simulink library "tqd"  (R2021b)
settings: Solver=VariableStepAuto  StartTime=0.0  StopTime=10.0  RelTol=1e-3
undefined symbols (not defined in the file): ATQD_AfterTqMinGain_X_Deg, ATQD_APSCreepBaseTqD_X_kph, ATQD_APSCreepBaseTqD_Y_Deg, ATQD_APSCreepBaseTqR_X_kph, ATQD_APSCreepBaseTqR_Y_Deg, ATQD_APSCreepIterm_X_kph, ATQD_APSCreepIterm_Y_kph, ATQD_APSCreepPterm_X_kph, ATQD_APSCreepPterm_Y_kph, ATQD_APSDecReq_X_kph, ATQD_APSDecReq_Y_mps2, ATQD_APSDecReqCMD_X_kph, ATQD_APSDecReqTs_X_pct, ATQD_APSDecTimeGain_X_Deg, ATQD_APSDecTimeGain_Y_s, ATQD_APSReqLowSpd_X_Deg, ATQD_AutoHoldReleaseBPS_X_Deg, ATQD_AWDLoadTrqnsGain_X_kg, ATQD_AWDLoadTrqnsGain_Y_pct, ATQD_BOSEnBPSPosn_X_kph, ATQD_BOSMap_X_rpm, ATQD_BOSMap_Y_pct, ATQD_CreepBaseTqD_X_kph, ATQD_CreepBaseTqD_Y_Deg, ATQD_CreepBaseTqR_X_kph, ATQD_CreepBaseTqR_Y_Deg, ATQD_CreepBPSDisPosn_X_Deg, ATQD_CreepBPSDisPosnR_X_Deg, ATQD_CreepBPSEnPosn_X_Deg, ATQD_CreepBPSEnPosnR_X_Deg, ATQD_CreepDeltaTq_X_kph, ATQD_CreepIterm_X_kph, ATQD_CreepIterm_Y_kph, ATQD_CreepItermMaxLimit_X_pct, ATQD_CreepPreloadTime_X_kph, ATQD_CreepPreloadTq_X_kph, ATQD_CreepPreloadTq_Y_s, ATQD_CreepProtTq_X_Deg, ATQD_CreepPterm_X_kph, ATQD_CreepPterm_Y_kph, ATQD_CreepRrTqSpRat_X_rpm, ATQD_CreepRrTqSpRat_Y_Nm, ATQD_CreepTargetSpdD_X_pct, ATQD_CreepTargetSpdR_X_pct, ATQD_ECOTqMapD_X_rpm, ATQD_ECOTqMapD_Y_pct, ATQD_EMTqMapD_X_rpm, ATQD_EMTqMapD_Y_pct, ATQD_EOPDTqMapDCon_X_rpm, ATQD_EOPDTqMapDCon_Y_Deg, ATQD_EscapeModePedTq_X_pct, ATQD_EscapeModePedTq_Y_rpm, ATQD_EscapeModePedTqFr_X_pct, ATQD_EscapeModePedTqFr_Y_rpm, ATQD_EstInitVehWeight_X_c, ATQD_FAfterTqCMDGain_X_rpm, ATQD_FAfterTqCMDGain_Y_pct, ATQD_FrLossMAPLowV_X_rpm, ATQD_FrLossMAPLowV_Y_Nm, ATQD_FrMotActReduce_X_rpm ... (+772)
libraries: simulink x211, hcu_lib x179, tqr x3
(part 17 of 28)

== system tqd/TQD/TorqueDemand/TorqueModule/TqDistribution/New Torque Distribution ==
  note: Torque Distribution Calculation
  note: Fr/Rr Wheel Torqrue Determination
  note: Motor Output Torque Status Determination
  note: Rr/Fr Motor Enable Output Torque Detection
  VPMM_DrivetrainSelect_enum : Inport
  VTQD_CoordTqDem_Nm : Inport  Port=2
  VTQR_NoABSFEDUWhlTqReq_Nm : Inport  Port=3
  VTQR_FrTqZeroTransLowBound_Nm : Inport  Port=4
  VTQR_NoABSREDUWhlTqReq_Nm : Inport  Port=5
  VTQR_RrTqZeroTransUpBound_Nm : Inport  Port=6
  VINP_RrMotorAvailTq_Nm : Inport  Port=7
  VINP_RrRegenAvailTq_Nm : Inport  Port=8
  VINP_FrMotorAvailTq_Nm : Inport  Port=9
  VINP_FrRegenAvailTq_Nm : Inport  Port=10
  VTQD_RrPreloadTq_Nm : Inport  Port=11
  VTQD_FrPreloadTq_Nm : Inport  Port=12
  VTQD_PreLoadHold_flg : Inport  Port=13
  AND{,1..8} (9 alike) : Logic  AllPortsSameDT=off  OutDataTypeStr=boolean
  Abs{,1..3} (4 alike) : Abs
  Add : Sum
  Add{1..3,5} (4 alike) : Sum  Inputs=+-
  Add4 : Sum
  Constant{1..2,21,49} (4 alike) : Constant  Value=KTQD_TqDemEnRrTMOutpRgn_Nm
  Constant10 : Constant  Value=KTQD_TqDemEnFrTMOutpMotDev_Nm
  Constant11 : Constant  Value=TRUE
  Constant12 : Constant  Value=ENUM_DRIVETRAIN_AWD
  Constant13 : Constant  Value=TRUE
  Constant14 : Constant  Value=ENUM_DRIVETRAIN_FWD
  Constant{15,18,30,39} (4 alike) : Constant  Value=ENUM_TMENOUTPTQSTA_REAR
  Constant{16,24,31,38} (4 alike) : Constant  Value=ENUM_TMENOUTPTQSTA_FRONT
  Constant{17,19,25,35,43} (5 alike) : Constant  Value=ENUM_TMENOUTPTQSTA_BOTH
  Constant{20,22..23,26..28,33,41,51} (9 alike) : Constant  Value=ZERO_FLOAT
  Constant29 : Constant  Value=EPS
  Constant3 : Constant  Value=KTQD_TqDemEnRrTMOutpRgnDev_Nm
  Constant{32,36,40,44} (4 alike) : Constant  Value=KTQD_NewDistInitRate_rat
  Constant34 : Constant  Value=ONE_FLOAT
  Constant37 : Constant  Value=EPS
  Constant4 : Constant  Value=KTQD_TqDemEnRrTMOutpMot_Nm
  Constant42 : Constant  Value=ONE_FLOAT
  Constant45 : Constant  Value=KTQD_AWDRrRatio_rat_ovrdflg
  Constant46 : Constant  Value=KTQD_AWDRrRatio_rat_ovrdval
  Constant47 : Constant  Value=KTQD_AWDRrRatio_rat_ovrdflg
  Constant48 : Constant  Value=KTQD_AWDRrRatio_rat_ovrdval
  Constant5 : Constant  Value=KTQD_TqDemEnFrTMOutpRgn_Nm
  Constant50 : Constant  Value=KTQD_TqDemEnRrTMOutpRgnDev_Nm
  Constant6 : Constant  Value=ENUM_DRIVETRAIN_AWD
  Constant7 : Constant  Value=ENUM_DRIVETRAIN_RWD
  Constant8 : Constant  Value=KTQD_RrTMRgnOutpConSW_flg
  Constant9 : Constant  Value=KTQD_FrTMMotOutpConSW_flg
  Delay : Delay  DelayLength=1  InitialCondition=uint8(0)
      settings: AttributesFormatString=%<InitialCondition>
  Divide : Product  Inputs=*/
  Divide1 : Product  Inputs=*/
  Equal{,1..9} (10 alike) : RelationalOperator  Operator===  OutDataTypeStr=boolean  RndMeth=Simplest
  KTQD_FrTMTotalGearRatio_gain{,1..4} (5 alike) : Gain  Gain=KTQD_FrTMTotalGearRatio_gain
  KTQD_RrTMTotalGearRatio_gain{,1..5} (6 alike) : Gain  Gain=KTQD_RrTMTotalGearRatio_gain
  Max : MinMax  Function=max  Inputs=2
  Max1 : MinMax  Function=max  Inputs=2
  Min : MinMax  Inputs=2
  Min1 : MinMax  Function=max  Inputs=2
  NOT : Logic  Operator=NOT  AllPortsSameDT=off  OutDataTypeStr=boolean
  NOT2 : Logic  Operator=NOT  AllPortsSameDT=off  OutDataTypeStr=boolean
  OR{,1..7} (8 alike) : Logic  Operator=OR  AllPortsSameDT=off  OutDataTypeStr=boolean
  Relational Operator{,5,8..9,12..13,16} (7 alike) : RelationalOperator  OutDataTypeStr=boolean  RndMeth=Simplest
  Relational Operator1 : RelationalOperator  Operator=<  OutDataTypeStr=boolean  RndMeth=Simplest
  Relational Operator{3..4,10..11} (4 alike) : RelationalOperator  Operator===  OutDataTypeStr=boolean  RndMeth=Simplest
  Relational Operator{2,7,14..15} (4 alike) : RelationalOperator  Operator=<=  OutDataTypeStr=boolean  RndMeth=Simplest
  Relational Operator6 : RelationalOperator  Operator=<  OutDataTypeStr=boolean  RndMeth=Simplest
  Saturation : Saturate  UpperLimit=single(1)  LowerLimit=single(0)
      settings: AttributesFormatString=|
      | UpperLimit:%<UpperLimit>
      | LowerLimi:%<LowerLimit>
  Saturation Dynamic : simulink/Discontinuities/Saturation Dynamic  OutMin=[]  OutMax=[]  OutDataTypeStr=Inherit: Same as second input  OutDataType=fixdt(1, 16)  OutScaling=2^-10  DoSatur=off
  Saturation Dynamic1 : simulink/Discontinuities/Saturation Dynamic  OutMin=[]  OutMax=[]  OutDataTypeStr=Inherit: Same as second input  OutDataType=fixdt(1, 16)  OutScaling=2^-10  DoSatur=off
  Saturation Dynamic2 : simulink/Discontinuities/Saturation Dynamic  OutMin=[]  OutMax=[]  OutDataTypeStr=Inherit: Same as second input  OutDataType=fixdt(1, 16)  OutScaling=2^-10  DoSatur=off
  Saturation1 : Saturate  UpperLimit=single(1)  LowerLimit=single(0)
      settings: AttributesFormatString=|
      | UpperLimit:%<UpperLimit>
      | LowerLimi:%<LowerLimit>
  Switch{,1..21} (22 alike) : Switch  Criteria=u2 ~= 0
      settings: AttributesFormatString=%<Criteria>
  VTQD_TMEnOutpTqSta_enum : Outport
  VTQD_NewDistFrWhlTq_Nm : Outport  Port=2
  VTQD_NewDistRrWhlTq_Nm : Outport  Port=3
  VTQD_NewFrRatio_rat : Outport  Port=4
  VTQD_NewRrRatio_rat : Outport  Port=5
  wires:
  [VTQD_CoordTqDem_Nm] -> Add5/1
  Saturation Dynamic2/1 -> Switch21/3
  [VTQD_CoordTqDem_Nm] -> Add3/1
  Equal9/1 -> Switch17/2
  [VTQD_PreLoadHold_flg] -> Switch10/2
  Constant14/1 -> Relational Operator11/2
  NOT/1 -> AND6/2
  VTQD_FrPreloadTq_Nm/1 -> [VTQD_FrPreloadTq_Nm]
  Constant42/1 -> Switch16/1
  Relational Operator16/1 -> Switch21/2
  Constant12/1 -> Relational Operator10/2
  Constant41/1 -> Switch15/1
  Constant38/1 -> Equal7/2
  Constant10/1 -> Add1/2
  Abs/1 -> Max/1
  Switch17/1 -> Switch18/3
  Constant34/1 -> Switch12/1
  AND3/1 -> OR2/1
  Switch10/1 -> [VTQD_NewDistFrWhlTq_Nm]  "VTQD_NewDistFrWhlTq_Nm"
  Equal8/1 -> Switch15/2
  Equal3/1 -> OR5/2
  Relational Operator6/1 -> AND3/1
  [VTQD_FrPreloadTq_Nm] -> Switch10/1
  Constant8/1 -> Switch/2
  Constant1/1 -> Relational Operator1/2
  Constant40/1 -> Switch15/3
  [VTQD_PreLoadHold_flg] -> Switch18/2
  [VTQD_NewFrRatio_rat] -> VTQD_NewFrRatio_rat/1
  Constant31/1 -> Equal5/2
  Constant4/1 -> Relational Operator/2
  AND4/1 -> OR2/2
  Constant44/1 -> Switch18/1
  Constant48/1 -> Switch20/1
  Constant39/1 -> Equal8/2
  Equal1/1 -> OR4/2
  OR2/1 -> AND5/2
  OR6/1 -> Switch/3
  Saturation1/1 -> Switch17/1
  Switch11/1 -> Switch12/3
  [VTQR_NoABSFEDUWhlTqReq_Nm] -> Relational Operator2/1
  Constant2/1 -> Add/1
  OR3/1 -> [VTQD_FrTMEnOutpTq_flg]  "VTQD_FrTMEnOutpTq_flg"
  Constant43/1 -> Equal9/2
  [VTQD_CoordTqDem_Nm] -> Relational Operator1/1
  Switch16/1 -> Switch17/3
  VPMM_DrivetrainSelect_enum/1 -> [VPMM_DrivetrainSelect_enum]
  KTQD_RrTMTotalGearRatio_gain5/1 -> Saturation Dynamic2/3
  Switch15/1 -> Switch16/3
  [VTQD_TMEnOutpTqSta_enum] -> Equal9/1
  VINP_FrRegenAvailTq_Nm/1 -> [VINP_FrRegenAvailTq_Nm]
  Constant28/1 -> Saturation Dynamic1/3
  VINP_RrMotorAvailTq_Nm/1 -> [VINP_RrMotorAvailTq_Nm]
  Relational Operator3/1 -> AND1/1
  Abs2/1 -> Max1/1
  [VINP_RrMotorAvailTq_Nm] -> KTQD_RrTMTotalGearRatio_gain1/1
  Max1/1 -> Divide1/2
  Equal7/1 -> Switch16/2
  [VINP_FrRegenAvailTq_Nm] -> KTQD_FrTMTotalGearRatio_gain4/1
  [VTQD_TMEnOutpTqSta_enum] -> Equal5/1
  Abs3/1 -> Divide1/1
  [VTQD_CoordTqDem_Nm] -> Min1/1
  [VTQR_RrTqZeroTransUpBound_Nm] -> Relational Operator7/2
  Divide1/1 -> Saturation1/1
  Switch18/1 -> Switch20/3  "VTQD_InitNewFrRatio_rat"
  [VTQD_TMEnOutpTqSta_enum] -> Equal8/1
  [VINP_FrRegenAvailTq_Nm] -> KTQD_FrTMTotalGearRatio_gain2/1
  [VTQD_PreLoadHold_flg] -> Switch9/2
  [VTQD_CoordTqDem_Nm] -> Relational Operator/1
  Switch/1 -> AND/2
  Switch12/1 -> Switch13/3
  [VTQD_TMEnOutpTqSta_enum] -> Equal7/1
  AND6/1 -> Switch2/2
  Constant13/1 -> Switch/1
  [VTQD_NewDistFrWhlTq_Nm] -> Abs3/1
  [VTQD_CoordTqDem_Nm] -> Abs2/1
  Constant6/1 -> Relational Operator3/2
  Relational Operator5/1 -> AND2/2
  Constant37/1 -> Max1/2
  Switch20/1 -> [VTQD_NewFrRatio_rat]  "VTQD_NewFrRatio_rat"
  [VTQD_CoordTqDem_Nm] -> Relational Operator13/1
  VTQR_NoABSREDUWhlTqReq_Nm/1 -> [VTQR_NoABSREDUWhlTqReq_Nm]
  Switch14/1 -> Switch19/3  "VTQD_InitNewRrRatio_rat"
  Add/1 -> Relational Operator2/2
  Delay/1 -> Switch2/3
  Relational Operator7/1 -> AND3/2
  Constant45/1 -> Switch19/2
  [VTQD_TMEnOutpTqSta_enum] -> Equal4/1
  [VPMM_DrivetrainSelect_enum] -> Relational Operator10/1
  [VTQR_NoABSFEDUWhlTqReq_Nm] -> Relational Operator5/1
  Equal4/1 -> Switch12/2
  Equal/1 -> OR4/1
  AND1/1 -> OR1/2
  Constant7/1 -> Relational Operator4/2
  [VTQR_FrTqZeroTransLowBound_Nm] -> Relational Operator5/2
  Relational Operator/1 -> AND2/1
  AND/1 -> OR/2
  [VPMM_DrivetrainSelect_enum] -> Relational Operator4/1
  [VTQR_NoABSREDUWhlTqReq_Nm] -> Relational Operator7/1
  OR1/1 -> [VTQD_RrTMEnOutpTq_flg]  "VTQD_RrTMEnOutpTq_flg"
  [VTQR_NoABSREDUWhlTqReq_Nm] -> Relational Operator9/1
  [VTQD_FrTMEnOutpTq_flg] -> AND8/2
  AND5/1 -> OR3/2
  Relational Operator8/1 -> AND4/1
  [VINP_RrMotorAvailTq_Nm] -> KTQD_RrTMTotalGearRatio_gain/1
  Relational Operator9/1 -> Switch1/3
  [VTQD_TMEnOutpTqSta_enum] -> Equal2/1
  Constant11/1 -> Switch1/1
  Switch2/1 -> Switch3/3
  [VTQD_RrTMEnOutpTq_flg] -> NOT2/1
  Relational Operator15/1 -> OR7/2
  NOT2/1 -> AND7/1
  Constant17/1 -> Switch4/1
  VTQR_RrTqZeroTransUpBound_Nm/1 -> [VTQR_RrTqZeroTransUpBound_Nm]
  [VTQD_RrTMEnOutpTq_flg] -> AND6/1
  [VTQD_RrTMEnOutpTq_flg] -> AND8/1
  Equal5/1 -> Switch11/2
  [VTQD_TMEnOutpTqSta_enum] -> Equal/1
  OR/1 -> AND1/2
  AND2/1 -> OR/1
  Relational Operator2/1 -> OR6/1
  [VTQD_TMEnOutpTqSta_enum] -> Equal3/1
  Constant18/1 -> Equal/2
  AND7/1 -> Switch3/2
  [VTQD_CoordTqDem_Nm] -> Add2/1
  Constant9/1 -> Switch1/2
  Add1/1 -> Relational Operator9/2
  OR5/1 -> Switch7/2
  [VTQD_FrTMEnOutpTq_flg] -> NOT/1
  [VTQD_CoordTqDem_Nm] -> Relational Operator6/1
  Constant36/1 -> Switch14/1
  Switch3/1 -> Switch4/3
  Constant20/1 -> Relational Operator12/2
  Relational Operator11/1 -> OR3/1
  OR4/1 -> Switch5/2
  [VTQD_TMEnOutpTqSta_enum] -> Equal1/1
  AND8/1 -> Switch4/2
  [VINP_RrMotorAvailTq_Nm] -> KTQD_RrTMTotalGearRatio_gain2/1
  [VTQD_CoordTqDem_Nm] -> Relational Operator12/1
  Add2/1 -> Saturation Dynamic/2
  Constant25/1 -> Equal3/2
  KTQD_RrTMTotalGearRatio_gain/1 -> Add1/1
  Relational Operator12/1 -> Switch6/2
  [VTQD_TMEnOutpTqSta_enum] -> Equal6/1
  [VTQD_CoordTqDem_Nm] -> Min/1
  KTQD_RrTMTotalGearRatio_gain2/1 -> Min/2
  Switch6/1 -> Switch5/1
  Constant51/1 -> Saturation Dynamic2/1
  Constant35/1 -> Equal6/2
  Switch4/1 -> Delay/1, [VTQD_TMEnOutpTqSta_enum]  "VTQD_TMEnOutpTqSta_enum"
  Min/1 -> Switch6/1
  [VPMM_DrivetrainSelect_enum] -> Relational Operator11/1
  Constant3/1 -> Add/2
  Equal2/1 -> OR5/1
  [VINP_RrMotorAvailTq_Nm] -> KTQD_RrTMTotalGearRatio_gain4/1
  VINP_FrMotorAvailTq_Nm/1 -> [VINP_FrMotorAvailTq_Nm]
  VTQR_FrTqZeroTransLowBound_Nm/1 -> [VTQR_FrTqZeroTransLowBound_Nm]
  Relational Operator4/1 -> OR1/1
  KTQD_FrTMTotalGearRatio_gain4/1 -> Relational Operator16/1
  Min1/1 -> Switch8/3
  Constant26/1 -> Switch7/3
  KTQD_RrTMTotalGearRatio_gain4/1 -> Add3/2
  [VTQD_CoordTqDem_Nm] -> Relational Operator8/1
  [VINP_FrMotorAvailTq_Nm] -> KTQD_FrTMTotalGearRatio_gain1/1
  KTQD_FrTMTotalGearRatio_gain/1 -> Min1/2
  [VTQR_NoABSFEDUWhlTqReq_Nm] -> Relational Operator14/1
  Relational Operator13/1 -> Switch8/2
  Switch9/1 -> [VTQD_NewDistRrWhlTq_Nm]  "VTQD_NewDistRrWhlTq_Nm"
  Switch7/1 -> Switch10/3
  Switch5/1 -> Switch9/3
  [VPMM_DrivetrainSelect_enum] -> Relational Operator3/1
  Add3/1 -> Saturation Dynamic1/2
  Switch8/1 -> Switch7/1
  [VINP_RrRegenAvailTq_Nm] -> KTQD_RrTMTotalGearRatio_gain3/1
  KTQD_FrTMTotalGearRatio_gain2/1 -> Relational Operator15/2
  Constant5/1 -> Relational Operator6/2
  Constant16/1 -> Switch3/1
  Constant46/1 -> Switch19/1
  [VTQD_CoordTqDem_Nm] -> Abs/1
  [VTQD_RrPreloadTq_Nm] -> Switch9/1
  Constant27/1 -> Relational Operator13/2
  Max/1 -> Divide/2
  KTQD_RrTMTotalGearRatio_gain3/1 -> Saturation Dynamic/3
  Constant29/1 -> Max/2
  KTQD_FrTMTotalGearRatio_gain1/1 -> Saturation Dynamic1/1
  [VTQD_FrTMEnOutpTq_flg] -> AND7/2
  Constant19/1 -> Equal1/2
  Divide/1 -> Saturation/1
  Switch1/1 -> AND4/2
  Abs1/1 -> Divide/1
  Constant32/1 -> Switch11/3
  Relational Operator10/1 -> AND5/1
  [VINP_FrRegenAvailTq_Nm] -> Add4/1
  KTQD_RrTMTotalGearRatio_gain1/1 -> Relational Operator8/2
  Constant22/1 -> Switch5/3
  Saturation Dynamic1/1 -> Switch8/1
  [VTQD_NewDistRrWhlTq_Nm] -> Abs1/1
  Constant30/1 -> Equal4/2
  Constant23/1 -> Saturation Dynamic/1
  Constant33/1 -> Switch11/1
  Constant24/1 -> Equal2/2
  [VINP_FrRegenAvailTq_Nm] -> KTQD_FrTMTotalGearRatio_gain3/1
  [VINP_FrRegenAvailTq_Nm] -> KTQD_FrTMTotalGearRatio_gain/1
  Saturation/1 -> Switch13/1
  Add5/1 -> Saturation Dynamic2/2
  [VTQD_NewRrRatio_rat] -> VTQD_NewRrRatio_rat/1
  Constant15/1 -> Switch2/1
  Equal6/1 -> Switch13/2
  [VTQD_PreLoadHold_flg] -> Switch14/2
  [VINP_RrRegenAvailTq_Nm] -> KTQD_RrTMTotalGearRatio_gain5/1
  Constant49/1 -> Add5/2
  Constant47/1 -> Switch20/2
  Switch13/1 -> Switch14/3
  [VTQD_CoordTqDem_Nm] -> Relational Operator15/1
  KTQD_FrTMTotalGearRatio_gain3/1 -> Add2/2
  Saturation Dynamic/1 -> Switch21/1
  Switch21/1 -> Switch6/3
  VTQD_PreLoadHold_flg/1 -> [VTQD_PreLoadHold_flg]
  VINP_RrRegenAvailTq_Nm/1 -> [VINP_RrRegenAvailTq_Nm]
  Constant50/1 -> Add4/2
  Add4/1 -> Relational Operator14/2
  OR7/1 -> AND/1
  Relational Operator14/1 -> OR6/2
  Switch19/1 -> [VTQD_NewRrRatio_rat]  "VTQD_NewRrRatio_rat"
  VTQR_NoABSFEDUWhlTqReq_Nm/1 -> [VTQR_NoABSFEDUWhlTqReq_Nm]
  [VTQD_NewDistFrWhlTq_Nm] -> VTQD_NewDistFrWhlTq_Nm/1
  VTQD_RrPreloadTq_Nm/1 -> [VTQD_RrPreloadTq_Nm]
  Relational Operator1/1 -> OR7/1
  [VTQD_NewDistRrWhlTq_Nm] -> VTQD_NewDistRrWhlTq_Nm/1
  Constant21/1 -> Relational Operator16/2
  [VTQD_TMEnOutpTqSta_enum] -> VTQD_TMEnOutpTqSta_enum/1
  VTQD_CoordTqDem_Nm/1 -> [VTQD_CoordTqDem_Nm]

== system tqd/TQD/TorqueDemand/TorqueModule/TqDistribution/RWD_Ratio ==
  Action Port : ActionPort
  Constant : Constant  Value=ONE_FLOAT
  Constant1 : Constant  Value=ZERO_FLOAT
  VTQD_FrRatio_RWD : Outport
  VTQD_RrRatio_RWD : Outport  Port=2
  wires:
  Constant1/1 -> VTQD_FrRatio_RWD/1
  Constant/1 -> VTQD_RrRatio_RWD/1

== system tqd/TQD/TorqueDemand/Signal_convert/SWC2_Subsystem/Big Mike Combo/Combo Key Detection ==
  TASK_TIME_10_MS : Inport
  VSCP_ComboKeyEn_flg : Inport  Port=2
  VSCP_ComboKeyReset_flg : Inport  Port=3
  VSCP_ComboKey_enum : Inport  Port=4
  VSCP_ComboKeyEnter_flg : Inport  Port=5
  VSCP_StreetFightModeOff_flg : Inport  Port=6
  DiagnosisOff Mode : Subsystem
  Engineering Mode : Subsystem
  Exhibition Mode : Subsystem
  Manufacture Mode : Subsystem
  Street Fight Mode : Subsystem
  VSCP_StreetFightMode_flg : Outport
  VSCP_EngineeringMode_flg : Outport  Port=2
  VSCP_ManufactureMode_flg : Outport  Port=3
  VSCP_ExhibitionMode_flg : Outport  Port=4
  VSCP_DiagnosisOffMode_flg : Outport  Port=5
  wires:
  [VSCP_DiagnosisOffMode_flg] -> VSCP_DiagnosisOffMode_flg/1
  DiagnosisOff Mode/1(VSCP_DiagnosisOffMode_flg) -> [VSCP_DiagnosisOffMode_flg]
  [VSCP_ComboKey_enum] -> DiagnosisOff Mode/4(VSCP_ComboKey_enum)
  [VSCP_ComboKeyEnter_flg] -> DiagnosisOff Mode/5(VSCP_ComboKeyEnter_flg)
  [TASK_TIME_10_MS] -> DiagnosisOff Mode/1(TASK_TIME_10_MS)
  [VSCP_ComboKeyReset_flg] -> DiagnosisOff Mode/3(VSCP_ComboKeyReset_flg)
  [VSCP_StreetFightModeOff_flg] -> DiagnosisOff Mode/6(VSCP_StreetFightModeOff_flg)
  [VSCP_ComboKeyEn_flg] -> DiagnosisOff Mode/2(VSCP_ComboKeyEn_flg)
  [VSCP_ExhibitionMode_flg] -> VSCP_ExhibitionMode_flg/1
  [VSCP_ManufactureMode_flg] -> VSCP_ManufactureMode_flg/1
  Exhibition Mode/1(VSCP_ExhibitionMode_flg) -> [VSCP_ExhibitionMode_flg]
  [VSCP_ComboKeyEn_flg] -> Exhibition Mode/2(VSCP_ComboKeyEn_flg)
  [VSCP_StreetFightModeOff_flg] -> Exhibition Mode/6(VSCP_StreetFightModeOff_flg)
  [VSCP_ComboKeyReset_flg] -> Exhibition Mode/3(VSCP_ComboKeyReset_flg)
  [TASK_TIME_10_MS] -> Exhibition Mode/1(TASK_TIME_10_MS)
  [VSCP_ComboKeyEnter_flg] -> Exhibition Mode/5(VSCP_ComboKeyEnter_flg)
  [VSCP_ComboKey_enum] -> Exhibition Mode/4(VSCP_ComboKey_enum)
  Manufacture Mode/1(VSCP_ManufactureMode_flg) -> [VSCP_ManufactureMode_flg]
  [VSCP_ComboKey_enum] -> Manufacture Mode/4(VSCP_ComboKey_enum)
  [VSCP_ComboKeyEnter_flg] -> Manufacture Mode/5(VSCP_ComboKeyEnter_flg)
  [TASK_TIME_10_MS] -> Manufacture Mode/1(TASK_TIME_10_MS)
  [VSCP_ComboKeyReset_flg] -> Manufacture Mode/3(VSCP_ComboKeyReset_flg)
  [VSCP_StreetFightModeOff_flg] -> Manufacture Mode/6(VSCP_StreetFightModeOff_flg)
  [VSCP_ComboKeyEn_flg] -> Manufacture Mode/2(VSCP_ComboKeyEn_flg)
  [VSCP_EngineeringMode_flg] -> VSCP_EngineeringMode_flg/1
  [VSCP_StreetFightMode_flg] -> VSCP_StreetFightMode_flg/1
  [VSCP_ComboKeyEn_flg] -> Engineering Mode/2(VSCP_ComboKeyEn_flg)
  [VSCP_StreetFightModeOff_flg] -> Engineering Mode/6(VSCP_StreetFightModeOff_flg)
  Engineering Mode/1(VSCP_EngineeringMode_flg) -> [VSCP_EngineeringMode_flg]
  [VSCP_ComboKeyReset_flg] -> Engineering Mode/3(VSCP_ComboKeyReset_flg)
  [TASK_TIME_10_MS] -> Engineering Mode/1(TASK_TIME_10_MS)
  [VSCP_ComboKeyEnter_flg] -> Engineering Mode/5(VSCP_ComboKeyEnter_flg)
  [VSCP_ComboKey_enum] -> Engineering Mode/4(VSCP_ComboKey_enum)
  VSCP_StreetFightModeOff_flg/1 -> [VSCP_StreetFightModeOff_flg]
  VSCP_ComboKeyEnter_flg/1 -> [VSCP_ComboKeyEnter_flg]
  VSCP_ComboKey_enum/1 -> [VSCP_ComboKey_enum]
  VSCP_ComboKeyReset_flg/1 -> [VSCP_ComboKeyReset_flg]
  VSCP_ComboKeyEn_flg/1 -> [VSCP_ComboKeyEn_flg]
  TASK_TIME_10_MS/1 -> [TASK_TIME_10_MS]
  [VSCP_ComboKey_enum] -> Street Fight Mode/4(VSCP_ComboKey_enum)
  [VSCP_ComboKeyEnter_flg] -> Street Fight Mode/5(VSCP_ComboKeyEnter_flg)
  [TASK_TIME_10_MS] -> Street Fight Mode/1(TASK_TIME_10_MS)
  [VSCP_ComboKeyReset_flg] -> Street Fight Mode/3(VSCP_ComboKeyReset_flg)
  Street Fight Mode/1(VSCP_StreetFightMode_flg) -> [VSCP_StreetFightMode_flg]
  [VSCP_StreetFightModeOff_flg] -> Street Fight Mode/6(VSCP_StreetFightModeOff_flg)
  [VSCP_ComboKeyEn_flg] -> Street Fight Mode/2(VSCP_ComboKeyEn_flg)

== system tqd/TQD/TorqueDemand/Signal_convert/SWC2_Subsystem/Big Mike Combo/Mode Coordination ==
  VSCP_StreetFightMode_flg : Inport
  VSCP_EngineeringMode_flg : Inport  Port=2
  VSCP_ManufactureMode_flg : Inport  Port=3
  VSCP_ExhibitionMode_flg : Inport  Port=4
  VSCP_DiagnosisOffMode_flg : Inport  Port=5
  DiagnosisOff : Subsystem  TreatAsAtomicUnit=on
  Engineering : Subsystem  TreatAsAtomicUnit=on
  Exhibition : Subsystem  TreatAsAtomicUnit=on
  If : If  NumInputs=5  IfExpression=u1 ~=0  ElseIfExpressions=u2 ~= 0, u3 ~= 0, u4 ~= 0, u5 ~= 0
  Manufacture : Subsystem  TreatAsAtomicUnit=on
  Merge : Merge  Inputs=6
  Product : Subsystem  TreatAsAtomicUnit=on
  StreetFight : Subsystem  TreatAsAtomicUnit=on
  VSCP_SysMode_enum : Outport
  wires:
  [VSCP_SysMode_enum] -> VSCP_SysMode_enum/1
  Merge/1 -> [VSCP_SysMode_enum]  "VTQD_SysMode_enum"
  Product/1(Product) -> Merge/6
  DiagnosisOff/1(DiagnosisOff) -> Merge/5
  Exhibition/1(Exhibition) -> Merge/4
  Manufacture/1(Manufacture) -> Merge/3
  Engineering/1(Engineering) -> Merge/2
  StreetFight/1(StreetFight) -> Merge/1
  If/5 -> DiagnosisOff/Action
  If/4 -> Exhibition/Action
  If/3 -> Manufacture/Action
  If/6 -> Product/Action
  If/2 -> Engineering/Action
  If/1 -> StreetFight/Action
  VSCP_DiagnosisOffMode_flg/1 -> [VSCP_DiagnosisOffMode_flg]
  VSCP_ExhibitionMode_flg/1 -> [VSCP_ExhibitionMode_flg]
  VSCP_ManufactureMode_flg/1 -> [VSCP_ManufactureMode_flg]
  VSCP_EngineeringMode_flg/1 -> [VSCP_EngineeringMode_flg]
  VSCP_StreetFightMode_flg/1 -> [VSCP_StreetFightMode_flg]
  [VSCP_EngineeringMode_flg] -> If/2
  [VSCP_ExhibitionMode_flg] -> If/4
  [VSCP_DiagnosisOffMode_flg] -> If/5
  [VSCP_StreetFightMode_flg] -> If/1
  [VSCP_ManufactureMode_flg] -> If/3

== system tqd/TQD/TorqueDemand/Signal_convert/SWC2_Subsystem/Big Mike Combo/Operation Condition ==
  VINP_PwrSta_enum : Inport
  VINP_ShiftGearPosn_enum : Inport  Port=2
  VSCP_ComboKeyEnCMD_flg : Inport  Port=3
  AND : Logic  AllPortsSameDT=off  OutDataTypeStr=boolean
  AND1 : Logic  AllPortsSameDT=off  OutDataTypeStr=boolean
  Constant1 : Constant  Value=ENUM_POWERSTA_ON
  Constant2 : Constant  Value=ENUM_POWERSTA_READY
  Constant3 : Constant  Value=ENUM_GEARPOSNTOCAN_N
  Constant4 : Constant  Value=ENUM_GEARPOSNTOCAN_P
  Equal{,1..3} (4 alike) : RelationalOperator  Operator===  OutDataTypeStr=boolean  RndMeth=Simplest
  OR : Logic  Operator=OR  AllPortsSameDT=off  OutDataTypeStr=boolean
  OR1 : Logic  Operator=OR  AllPortsSameDT=off  OutDataTypeStr=boolean
  VSCP_ComboKeyPreEn_flg : Outport
  VSCP_ComboKeyEn_flg : Outport  Port=2
  wires:
  [VSCP_ComboKeyEn_flg] -> VSCP_ComboKeyEn_flg/1
  AND1/1 -> [VSCP_ComboKeyEn_flg]  "VTQD_ComboKeyEn_flg"
  [VSCP_ComboKeyEnCMD_flg] -> AND1/2
  [VSCP_ComboKeyPreEn_flg] -> AND1/1
  VSCP_ComboKeyEnCMD_flg/1 -> [VSCP_ComboKeyEnCMD_flg]
  AND/1 -> [VSCP_ComboKeyPreEn_flg]  "VTQD_ComboKeyPreEn_flg"
  [VSCP_ComboKeyPreEn_flg] -> VSCP_ComboKeyPreEn_flg/1
  VINP_ShiftGearPosn_enum/1 -> [VINP_ShiftGearPosn_enum]
  VINP_PwrSta_enum/1 -> [VINP_PwrSta_enum]
  OR1/1 -> AND/2
  Equal1/1 -> OR/2
  [VINP_PwrSta_enum] -> Equal1/1
  Constant2/1 -> Equal/2
  [VINP_PwrSta_enum] -> Equal/1
  [VINP_ShiftGearPosn_enum] -> Equal3/1
  Constant4/1 -> Equal2/2
  Equal3/1 -> OR1/2
  Constant1/1 -> Equal1/2
  [VINP_ShiftGearPosn_enum] -> Equal2/1
  Equal/1 -> OR/1
  Constant3/1 -> Equal3/2
  Equal2/1 -> OR1/1
  OR/1 -> AND/1

== system tqd/TQD/TorqueDemand/Signal_convert/SWC2_Subsystem/Big Mike Combo/Signal Status Detection ==
  note: Combo Key Note:
      | ENUM_COMBOKEY_NONE = uint8(0); None
      | ENUM_COMBOKEY_REGENDOWN = uint8(1); VINP_SWC2RegenDown_flg
      | ENUM_COMBOKEY_REGENUP = uint8(2); VINP_SWC2RegenUp_flg
      | ENUM_COMBOKEY_RESUP = uint8(3); VINP_SWC2LScrollUpSta_flg
      | ENUM_COMBOKEY_SETDOWN = uint8(4); VINP_SWC2LScrollDownSta_flg
      | ENUM_COMBOKEY_SWCUP = uint8(5); VINP_SWC2RScrollUpSta_flg
      | ENUM_COMBOKEY_SWCDOWN = uint8(6); VINP_SWC2RScrollDownSta_flg
      | ENUM_COMBOKEY_CANCEL = uint8(7); VINP_SWC2LScrollPressSta_flg
      | ENUM_COMBOKEY_SWCACC = uint8(8); VINP_SWC2LADASSta_flg
      | ENUM_COMBOKEY_DISTANCE = uint8(9); VINP_SWC2LDriveModeSta_flg
      | ENUM_COMBOKEY_SWCMODE = uint8(10); VINP_SWC2RScrollPressSta_flg
      | ENUM_COMBOKEY_SWCRIGHT = uint8(11); VINP_SWC2RRightSta_flg
      | ENUM_COMBOKEY_SWCLEFT = uint8(12); VINP_SWC2RLeftSta_flg
  TASK_TIME_10_MS : Inport
  VINP_SWCRegenDown_flg : Inport  Port=2
  VINP_SWCRegenUp_flg : Inport  Port=3
  VINP_SWCResUpSta_flg : Inport  Port=4
  VINP_SWCSetdownSta_flg : Inport  Port=5
  VINP_SWCUpSta_flg : Inport  Port=6
  VINP_SWCDownSta_flg : Inport  Port=7
  VINP_SWCCANCELSta_flg : Inport  Port=8
  VSCP_ComboKeyPreEn_flg : Inport  Port=9
  VINP_SWCACCSta_flg : Inport  Port=10
  VSCP_SysMode_enum : Inport  Port=11
  VINP_SWCDistanceSta_flg : Inport  Port=12
  VINP_SWCmodeSta_flg : Inport  Port=13
  VINP_SWCRightSta_flg : Inport  Port=14
  VINP_SWCLeftSta_flg : Inport  Port=15
  VSCP_ComboKeyEn_flg : Inport  Port=16
  AND{,1..14} (15 alike) : Logic  AllPortsSameDT=off  OutDataTypeStr=boolean
  Constant{,1..5,10..15} (12 alike) : Constant  Value=KTQD_SetSpdShortPLim_s
  Constant{6..9} (4 alike) : Constant  Value=KTQD_ComboKeyLongDet_s
  Delay : Delay  DelayLength=1
  DelayEnable{,1..15} (16 alike) : hcu_lib/Basic_Blocks/DelayEnable
  Detect Decrease{,1..15} (16 alike) : simulink/Logic and Bit Operations/Detect Decrease  vinit=0.0  OutDataTypeStr=boolean
  If : If  NumInputs=12  IfExpression=u1~=0  ElseIfExpressions=u2~=0,u3~=0,u4~=0,u5~=0,u6~=0,u7 ~=0,u8~=0,u9~=0,u10~=0,u11~=0,u12~=0
  Merge : Merge  Inputs=13
  None : Subsystem  TreatAsAtomicUnit=on
  SR_Latch : hcu_lib/Basic_Blocks/SR_Latch
  SWCACCSta : Subsystem  TreatAsAtomicUnit=on
  SWCCANCELStaShort : Subsystem  TreatAsAtomicUnit=on
  SWCDistanceSta : Subsystem  TreatAsAtomicUnit=on
  SWCDownStaShort : Subsystem  TreatAsAtomicUnit=on
  SWCLeftSta : Subsystem  TreatAsAtomicUnit=on
  SWCRegenDownShort : Subsystem  TreatAsAtomicUnit=on
  SWCRegenUpShort : Subsystem  TreatAsAtomicUnit=on
  SWCResUpStaShort : Subsystem  TreatAsAtomicUnit=on
  SWCRightSta : Subsystem  TreatAsAtomicUnit=on
  SWCSetdownStaShort : Subsystem  TreatAsAtomicUnit=on
  SWCUpStaShort : Subsystem  TreatAsAtomicUnit=on
  SWCmodeSta : Subsystem  TreatAsAtomicUnit=on
  Street Fight Switch Off : Subsystem
  VSCP_ComboKey_enum : Outport
  VSCP_ComboKeyEnCMD_flg : Outport  Port=2
  VSCP_ComboKeyReset_flg : Outport  Port=3
  VSCP_ComboKeyEnter_flg : Outport  Port=4
  VSCP_StreetFightModeOff_flg : Outport  Port=5
  wires:
  [VSCP_ComboKeyEn_flg] -> Delay/1
  Delay/1 -> AND8/2
  VSCP_ComboKeyEn_flg/1 -> [VSCP_ComboKeyEn_flg]
  [VSCP_SWCLeftSta_flg] -> AND14/1
  [VSCP_SWCRightSta_flg] -> AND13/1
  [VSCP_SWCmodeSta_flg] -> AND12/1
  [VSCP_SWCDistanceSta_flg] -> AND11/1
  [VSCP_SWCACCSta_flg] -> AND10/1
  [VSCP_SWCCANCELStaShort_flg] -> AND9/1
  [VSCP_SWCDownStaShort_flg] -> AND6/1
  [VSCP_SWCUpStaShort_flg] -> AND5/1
  [VSCP_SWCSetdownStaShort_flg] -> AND4/1
  [VSCP_SWCRegenUpShort_flg] -> AND2/1
  [VSCP_SWCRegenDownShort_flg] -> AND1/1
  [SWCLeftSta_enum] -> Merge/12
  [SWCRightSta_enum] -> Merge/11
  [SWCmodeSta_enum] -> Merge/10
  [SWCDistanceSta_enum] -> Merge/9
  [SWCACCSta_enum] -> Merge/8
  [SWCCANCELStaShort_enum] -> Merge/7
  [None_enum] -> Merge/13
  SWCLeftSta/1(SWCLeftSta_enum) -> [SWCLeftSta_enum]
  If/12 -> SWCLeftSta/Action
  AND14/1 -> If/12
  [VSCP_ComboKeyPreEn_flg] -> AND14/2
  [VINP_SWCLeftSta_flg] -> DelayEnable15/1
  [TASK_TIME_10_MS] -> DelayEnable15/3
  Constant15/1 -> DelayEnable15/2
  DelayEnable15/1 -> Detect Decrease15/1
  Detect Decrease15/1 -> [VSCP_SWCLeftSta_flg]  "VTQD_SWCLeftSta_flg"
  VINP_SWCLeftSta_flg/1 -> [VINP_SWCLeftSta_flg]
  SWCRightSta/1(SWCRightSta_enum) -> [SWCRightSta_enum]
  If/11 -> SWCRightSta/Action
  AND13/1 -> If/11
  [VSCP_ComboKeyPreEn_flg] -> AND13/2
  Detect Decrease14/1 -> [VSCP_SWCRightSta_flg]  "VTQD_SWCRightSta_flg"
  DelayEnable14/1 -> Detect Decrease14/1
  Constant14/1 -> DelayEnable14/2
  [TASK_TIME_10_MS] -> DelayEnable14/3
  [VINP_SWCRightSta_flg] -> DelayEnable14/1
  VINP_SWCRightSta_flg/1 -> [VINP_SWCRightSta_flg]
  SWCmodeSta/1(SWCmodeSta_enum) -> [SWCmodeSta_enum]
  If/10 -> SWCmodeSta/Action
  AND12/1 -> If/10
  [VSCP_ComboKeyPreEn_flg] -> AND12/2
  [VINP_SWCmodeSta_flg] -> DelayEnable13/1
  [TASK_TIME_10_MS] -> DelayEnable13/3
  Constant13/1 -> DelayEnable13/2
  DelayEnable13/1 -> Detect Decrease13/1
  Detect Decrease13/1 -> [VSCP_SWCmodeSta_flg]  "VTQD_SWCmodeSta_flg"
  VINP_SWCmodeSta_flg/1 -> [VINP_SWCmodeSta_flg]
  SWCDistanceSta/1(SWCDownStaShort_enum) -> [SWCDistanceSta_enum]
  If/9 -> SWCDistanceSta/Action
  AND11/1 -> If/9
  [VSCP_ComboKeyPreEn_flg] -> AND11/2
  Detect Decrease12/1 -> [VSCP_SWCDistanceSta_flg]  "VTQD_SWCDistanceSta_flg"
  DelayEnable12/1 -> Detect Decrease12/1
  Constant12/1 -> DelayEnable12/2
  [TASK_TIME_10_MS] -> DelayEnable12/3
  [VINP_SWCDistanceSta_flg] -> DelayEnable12/1
  VINP_SWCDistanceSta_flg/1 -> [VINP_SWCDistanceSta_flg]
  If/8 -> SWCACCSta/Action
  SWCACCSta/1(SWCACCSta_enum) -> [SWCACCSta_enum]
  AND10/1 -> If/8
  [VSCP_ComboKeyPreEn_flg] -> AND10/2
  If/7 -> SWCCANCELStaShort/Action
  SWCCANCELStaShort/1(SWCCANCELStaShort_enum) -> [SWCCANCELStaShort_enum]
  AND9/1 -> If/7
  [VSCP_ComboKeyPreEn_flg] -> AND9/2
  [VINP_SWCACCSta_flg] -> DelayEnable11/1
  [TASK_TIME_10_MS] -> DelayEnable11/3
  Constant11/1 -> DelayEnable11/2
  DelayEnable11/1 -> Detect Decrease11/1
  Detect Decrease11/1 -> [VSCP_SWCACCSta_flg]  "VTQD_SWCACCSta_flg"
  [VSCP_SysMode_enum] -> Street Fight Switch Off/5(VSCP_SysMode_enum)
  VSCP_SysMode_enum/1 -> [VSCP_SysMode_enum]
  [VSCP_StreetFightModeOff_flg] -> VSCP_StreetFightModeOff_flg/1
  [VSCP_SWCCANCELStaLong_flg] -> Street Fight Switch Off/4(SWCCANCELStaLong_flg)
  [VSCP_ComboKeyPreEn_flg] -> Street Fight Switch Off/3(VSCP_ComboKeyPreEn_flg)
  [VSCP_SWCCANCELStaShort_flg] -> Street Fight Switch Off/2(VSCP_SWCCANCELStaShort_flg)
  [TASK_TIME_10_MS] -> Street Fight Switch Off/1(TASK_TIME_10_MS)
  Street Fight Switch Off/1(VSCP_StreetFightModeOff_flg) -> [VSCP_StreetFightModeOff_flg]
  Detect Decrease10/1 -> [VSCP_SWCCANCELStaShort_flg]  "VTQD_SWCCANCELStaShort_flg"
  DelayEnable10/1 -> Detect Decrease10/1
  Constant10/1 -> DelayEnable10/2
  [TASK_TIME_10_MS] -> DelayEnable10/3
  [VINP_SWCCANCELSta_flg] -> DelayEnable10/1
  AND8/1 -> [VSCP_ComboKeyEnter_flg]  "VTQD_ComboKeyEnter_flg"
  Detect Decrease9/1 -> AND8/1
  AND7/1 -> [VSCP_ComboKeyReset_flg]  "VTQD_ComboKeyReset_flg"
  [VSCP_ComboKeyEn_flg] -> AND7/2
  Detect Decrease8/1 -> AND7/1
  [VSCP_ComboKeyEnter_flg] -> VSCP_ComboKeyEnter_flg/1
  [VSCP_SWCCANCELStaLong_flg] -> Detect Decrease9/1
  [VSCP_ComboKeyReset_flg] -> VSCP_ComboKeyReset_flg/1
  [VSCP_SWCACCStaLong_flg] -> Detect Decrease8/1
  VINP_SWCACCSta_flg/1 -> [VINP_SWCACCSta_flg]
  [VINP_SWCACCSta_flg] -> DelayEnable9/1
  [TASK_TIME_10_MS] -> DelayEnable9/3
  Constant9/1 -> DelayEnable9/2
  DelayEnable9/1 -> [VSCP_SWCACCStaLong_flg]  "VTQD_SWCACCStaLong_flg"
  [VSCP_ComboKeyPreEn_flg] -> AND6/2
  AND6/1 -> If/6
  [VSCP_ComboKeyPreEn_flg] -> AND5/2
  AND5/1 -> If/5
  [VSCP_ComboKeyPreEn_flg] -> AND4/2
  AND4/1 -> If/4
  [VSCP_ComboKeyPreEn_flg] -> AND3/2
  [VSCP_SWCResUpStaShort_flg] -> AND3/1
  AND3/1 -> If/3
  [VSCP_ComboKeyPreEn_flg] -> AND2/2
  AND2/1 -> If/2
  [VSCP_ComboKeyPreEn_flg] -> AND1/2
  AND1/1 -> If/1
  VSCP_ComboKeyPreEn_flg/1 -> [VSCP_ComboKeyPreEn_flg]
  Detect Decrease7/1 -> SR_Latch/2
  [VSCP_SWCCANCELStaLong_flg] -> Detect Decrease7/1
  Detect Decrease6/1 -> SR_Latch/1
  AND/1 -> Detect Decrease6/1
  [VSCP_ComboKeyEnCMD_flg] -> VSCP_ComboKeyEnCMD_flg/1
  DelayEnable8/1 -> [VSCP_SWCCANCELStaLong_flg]  "VTQD_SWCCANCELStaLong_flg"
  Constant8/1 -> DelayEnable8/2
  [TASK_TIME_10_MS] -> DelayEnable8/3
  [VINP_SWCCANCELSta_flg] -> DelayEnable8/1
  VINP_SWCCANCELSta_flg/1 -> [VINP_SWCCANCELSta_flg]
  SR_Latch/1 -> [VSCP_ComboKeyEnCMD_flg]  "VTQD_ComboKeyEnCMD_flg"
  [VSCP_SWCRegenUpLong_flg] -> AND/2
  [VSCP_SWCRegenDownLong_flg] -> AND/1
  [VINP_SWCRegenUp_flg] -> DelayEnable7/1
  [TASK_TIME_10_MS] -> DelayEnable7/3
  Constant7/1 -> DelayEnable7/2
  DelayEnable7/1 -> [VSCP_SWCRegenUpLong_flg]  "VTQD_SWCRegenUpLong_flg"
  DelayEnable6/1 -> [VSCP_SWCRegenDownLong_flg]  "VTQD_SWCRegenDownLong_flg"
  Constant6/1 -> DelayEnable6/2
  [TASK_TIME_10_MS] -> DelayEnable6/3
  [VINP_SWCRegenDown_flg] -> DelayEnable6/1
  SWCDownStaShort/1(SWCDownStaShort_enum) -> [SWCDownStaShort_enum]
  Merge/1 -> [VSCP_ComboKey_enum]  "VTQD_ComboKey_enum"
  SWCSetdownStaShort/1(SWCSetdownStaShort_enum) -> [SWCSetdownStaShort_enum]
  SWCResUpStaShort/1(SWCResUpStaShort_enum) -> [SWCResUpStaShort_enum]
  SWCRegenDownShort/1(SWCRegenDownShort_enum) -> [SWCRegenDownShort_enum]
  If/3 -> SWCResUpStaShort/Action
  DelayEnable1/1 -> Detect Decrease1/1
  [TASK_TIME_10_MS] -> DelayEnable1/3
  [VINP_SWCRegenUp_flg] -> DelayEnable1/1
  None/1(None_enum) -> [None_enum]
  [SWCRegenDownShort_enum] -> Merge/1
  VINP_SWCUpSta_flg/1 -> [VINP_SWCUpSta_flg]
  DelayEnable2/1 -> Detect Decrease2/1
  [TASK_TIME_10_MS] -> DelayEnable2/3
  [VINP_SWCResUpSta_flg] -> DelayEnable2/1
  DelayEnable/1 -> Detect Decrease/1
  VINP_SWCRegenUp_flg/1 -> [VINP_SWCRegenUp_flg]
  [SWCDownStaShort_enum] -> Merge/6
  [VINP_SWCRegenDown_flg] -> DelayEnable/1
  VINP_SWCSetdownSta_flg/1 -> [VINP_SWCSetdownSta_flg]
  [TASK_TIME_10_MS] -> DelayEnable/3
  Constant1/1 -> DelayEnable1/2
  If/1 -> SWCRegenDownShort/Action
  [SWCRegenUpShort_enum] -> Merge/2
  Constant4/1 -> DelayEnable4/2
  [VINP_SWCUpSta_flg] -> DelayEnable4/1
  VINP_SWCDownSta_flg/1 -> [VINP_SWCDownSta_flg]
  Detect Decrease1/1 -> [VSCP_SWCRegenUpShort_flg]  "VTQD_SWCRegenUpShort_flg"
  If/4 -> SWCSetdownStaShort/Action
  Detect Decrease2/1 -> [VSCP_SWCResUpStaShort_flg]  "VTQD_SWCResUpStaShort_flg"
  If/13 -> None/Action
  [TASK_TIME_10_MS] -> DelayEnable4/3
  TASK_TIME_10_MS/1 -> [TASK_TIME_10_MS]
  Detect Decrease/1 -> [VSCP_SWCRegenDownShort_flg]  "VTQD_SWCRegenDownShort_flg"
  If/5 -> SWCUpStaShort/Action
  [VINP_SWCDownSta_flg] -> DelayEnable5/1
  DelayEnable3/1 -> Detect Decrease3/1
  [SWCResUpStaShort_enum] -> Merge/3
  VINP_SWCRegenDown_flg/1 -> [VINP_SWCRegenDown_flg]
  Constant3/1 -> DelayEnable3/2
  [TASK_TIME_10_MS] -> DelayEnable5/3
  [SWCSetdownStaShort_enum] -> Merge/4
  [TASK_TIME_10_MS] -> DelayEnable3/3
  If/6 -> SWCDownStaShort/Action
  Constant5/1 -> DelayEnable5/2
  DelayEnable5/1 -> Detect Decrease5/1
  Detect Decrease4/1 -> [VSCP_SWCUpStaShort_flg]  "VTQD_SWCUpStaShort_flg"
  DelayEnable4/1 -> Detect Decrease4/1
  Constant2/1 -> DelayEnable2/2
  If/2 -> SWCRegenUpShort/Action
  Detect Decrease5/1 -> [VSCP_SWCDownStaShort_flg]  "VTQD_SWCDownStaShort_flg"
  Detect Decrease3/1 -> [VSCP_SWCSetdownStaShort_flg]  "VTQD_SWCSetdownStaShort_flg"
  SWCUpStaShort/1(SWCUpStaShort_enum) -> [SWCUpStaShort_enum]
  [VINP_SWCSetdownSta_flg] -> DelayEnable3/1
  VINP_SWCResUpSta_flg/1 -> [VINP_SWCResUpSta_flg]
  [SWCUpStaShort_enum] -> Merge/5
  SWCRegenUpShort/1(SWCRegenUpShort_enum) -> [SWCRegenUpShort_enum]
  Constant/1 -> DelayEnable/2
  [VSCP_ComboKey_enum] -> VSCP_ComboKey_enum/1

== system tqd/TQD/TorqueDemand/Signal_convert/SWC2_Subsystem/Speed Setting Mode/ACC Speed Setting ON ==
  note: ACCSetSpd_241018
  note: ACC SPEED SETTING Signal
  VTQD_SWC2ScrollUpSta_enum : Inport
  VTQD_SWC2ScrollDownSta_enum : Inport  Port=2
  VVMC_LVDAACCStatusInformation_flg : Inport  Port=3
  VVMC_ACCObjDist_m : Inport  Port=4
  VTQD_SpdLim4SetSpd_raw32 : Inport  Port=5
  VINP_ADASACCSta_enum : Inport  Port=6
  VINP_Distanceunit_flg : Inport  Port=7
  VINP_SmartEcoModeSW_flg : Inport  Port=8
  VVMC_SetACCDisableAPS_flg : Inport  Port=9
  VINP_IVIACCAdaptiveSta_flg : Inport  Port=10
  VTQD_Set2MeterSpd_flg : Inport  Port=11
  VTQD_SetRoadSpdLim_flg : Inport  Port=12
  VINP_ADASSLIFSpdLim_enum : Inport  Port=13
  VTQD_LScrollPressShort_flg : Inport  Port=14
  VVMC_MeterIndSpeed_raw32 : Inport  Port=15
  VTQD_SWC2ScrollDownSta_flg : Inport  Port=16
  VTQD_SWC2ScrollUpSta_flg : Inport  Port=17
  VTQD_LastSetSpd_kph : Inport  Port=18
  Action Port : ActionPort  InitializeStates=reset
  " 20" : Constant  Value=KTQD_ACCActiveMetSpdLoMPH_mph
  " 30kph" : Constant  Value=KTQD_ACCActiveMetSpdLo_kph
  0 : Constant  Value=KTQD_AllowSetSpdOvrd_flg
  1 : Constant  Value=KTQD_AllowSetSpdOvrdVal_flg
  105 : Constant  Value=KTQD_ACCActiveMetSpdHiMPH_mph
  10kph1 : Constant  Value=KTQD_AllowSetSpdSpd_kph
  180kph : Constant  Value=KTQD_ACCActiveMetSpdHi_kph
  2 : Constant  Value=KTQD_SmartEcoLimitSpd_kph
  2m : Constant  Value=KVMC_NotAllowSetSpdDist_m
  3 : Constant  Value=KTQD_SmartEcoLimitSpd_mph
  5 : Constant  Value=KTQD_SetSpdDeltaLongMPH_mph
  5kph : Constant  Value=KTQD_SetSpdDeltaLong_kph
  6m : Constant  Value=KVMC_AllowSetSpdDist_m
  ACCSetSpd_2506 : Stateflow chart  TreatAsAtomicUnit=on
  AND : Logic  AllPortsSameDT=off  OutDataTypeStr=boolean
  AND1 : Logic  AllPortsSameDT=off  OutDataTypeStr=boolean
  AND2 : Logic  AllPortsSameDT=off  OutDataTypeStr=boolean
  Cast To Single : DataTypeConversion  OutDataTypeStr=int8
  Constant126 : Constant  Value=0x0  OutDataTypeStr=uint8
  Equal53 : RelationalOperator  Operator=~=  OutDataTypeStr=boolean  RndMeth=Simplest
  ONE : Constant  Value=ONE_INT
  OR : Logic  Operator=OR  AllPortsSameDT=off  OutDataTypeStr=boolean
  Relational Operator : RelationalOperator  Operator=<=  OutDataTypeStr=boolean  RndMeth=Simplest
  Relational Operator1 : RelationalOperator  Operator=>  OutDataTypeStr=boolean  RndMeth=Simplest
  Relational Operator2 : RelationalOperator  Operator===  OutDataTypeStr=boolean  RndMeth=Simplest
  Relational Operator3 : RelationalOperator  OutDataTypeStr=boolean  RndMeth=Simplest
  Relational Operator4 : RelationalOperator  Operator===  OutDataTypeStr=boolean  RndMeth=Simplest
  Round : Rounding  Operator=round
  Switch{,1..6} (7 alike) : Switch  Criteria=u2 > Threshold
  Terminator : Terminator
  standby : Constant  Value=ENUM_ADASACCSTA_STANDBY
  zero : Constant  Value=ZERO_INT
  VTQD_ACCSetSpd_kph : Outport
  VTQD_SWC2AllowSetSpd_flg : Outport  Port=2
  wires:
  VVMC_LVDAACCStatusInformation_flg/1 -> [VVMC_LVDAACCStatusInformation_flg]
  Switch4/1 -> [VTQD_SetSpdDeltaLong_raw32]  "VTQD_SetSpdDeltaLong_raw32"
  Switch3/1 -> [VTQD_ACCActiveMetSpdLo_raw32]  "VTQD_ACCActiveMetSpdLo_raw32"
  VTQD_SpdLim4SetSpd_raw32/1 -> [VTQD_SpdLim4SetSpd_raw32]
  VINP_ADASACCSta_enum/1 -> [VINP_ADASACCSta_enum]
  6m/1 -> Relational Operator/2
  2m/1 -> Relational Operator1/2
  Relational Operator/1 -> AND/1
  Relational Operator1/1 -> AND/2
  [VVMC_MeterIndSpeed_raw32] -> Relational Operator3/1
  10kph1/1 -> Relational Operator3/2
  AND/1 -> OR/1
  Relational Operator3/1 -> OR/2
  Switch/1 -> Terminator/1, VTQD_SWC2AllowSetSpd_flg/1  "VTQD_SWC2AllowSetSpd_flg"
  OR/1 -> AND2/1
  0/1 -> Switch/2
  1/1 -> Switch/1
  Cast To Single/1 -> Relational Operator4/1, Switch1/3
  Switch1/1 -> VTQD_ACCSetSpd_kph/1
  [VINP_ADASACCSta_enum] -> Relational Operator2/1
  AND1/1 -> Switch1/2
  ONE/1 -> Switch1/1
  standby/1 -> Relational Operator2/2
  zero/1 -> Relational Operator4/2
  Relational Operator2/1 -> AND1/1
  Relational Operator4/1 -> AND1/2
  VINP_Distanceunit_flg/1 -> [VINP_Distanceunit_flg]
  [VINP_Distanceunit_flg] -> Switch2/2
  Switch2/1 -> [VTQD_ACCActiveMetSpdHi_raw32]  "VTQD_ACCActiveMetSpdHi_raw32"
  [VINP_Distanceunit_flg] -> Switch3/2
  " 30kph"/1 -> Switch3/3
  " 20"/1 -> Switch3/1
  [VINP_Distanceunit_flg] -> Switch4/2
  5kph/1 -> Switch4/3
  5/1 -> Switch4/1
  Round/1 -> Cast To Single/1
  VTQD_SWC2ScrollUpSta_enum/1 -> [VTQD_SWC2ScrollUpSta_enum]
  VINP_SmartEcoModeSW_flg/1 -> [VINP_SmartEcoModeSW_flg]
  180kph/1 -> Switch5/3
  [VINP_SmartEcoModeSW_flg] -> Switch5/2
  Switch5/1 -> Switch2/3
  [VINP_SmartEcoModeSW_flg] -> Switch6/2
  105/1 -> Switch6/3
  Switch6/1 -> Switch2/1
  3/1 -> Switch6/1
  2/1 -> Switch5/1
  AND2/1 -> Switch/3
  [VINP_ADASACCSta_enum] -> ACCSetSpd_2506/1(VINP_ADASACCSta_enum)
  [VTQD_SpdLim4SetSpd_raw32] -> ACCSetSpd_2506/3(VTQD_SpdLim4SetSpd_raw32)
  [VTQD_ACCActiveMetSpdHi_raw32] -> ACCSetSpd_2506/4(VTQD_ACCActiveMetSpdHi_raw32)
  [VTQD_ACCActiveMetSpdLo_raw32] -> ACCSetSpd_2506/5(VTQD_ACCActiveMetSpdLo_raw32)
  [VTQD_SWC2ScrollUpSta_enum] -> ACCSetSpd_2506/7(VTQD_SWC2ScrollUpSta_enum)
  [VTQD_SWC2ScrollDownSta_enum] -> ACCSetSpd_2506/8(VTQD_SWC2ScrollDownSta_enum)
  [VTQD_SetSpdDeltaLong_raw32] -> ACCSetSpd_2506/9(VTQD_SetSpdDeltaLong_raw32)
  [VINP_Distanceunit_flg] -> ACCSetSpd_2506/11(VINP_Distanceunit_flg)
  Constant126/1 -> Equal53/2
  ACCSetSpd_2506/1(VTQD_ACCSetSpd_raw32) -> [VTQD_ACCSetSpd_raw32]  "VTQD_ACCSetSpd_raw32"
  [VTQD_ACCSetSpd_raw32] -> Round/1
  [VVMC_LVDAACCStatusInformation_flg] -> ACCSetSpd_2506/14(VVMC_LVDAACCStatusInformation_flg)
  VTQD_SWC2ScrollDownSta_enum/1 -> [VTQD_SWC2ScrollDownSta_enum]
  VVMC_ACCObjDist_m/1 -> [VVMC_ACCObjDist_m]
  [VVMC_ACCObjDist_m] -> Relational Operator/1
  [VVMC_ACCObjDist_m] -> Relational Operator1/1
  VVMC_SetACCDisableAPS_flg/1 -> [VVMC_SetACCDisableAPS_flg]
  [VVMC_SetACCDisableAPS_flg] -> AND2/2
  VINP_IVIACCAdaptiveSta_flg/1 -> [VINP_IVIACCAdaptiveSta_flg]
  [VINP_IVIACCAdaptiveSta_flg] -> ACCSetSpd_2506/2(VINP_IVIACCAdaptiveSta_flg)
  VTQD_Set2MeterSpd_flg/1 -> [VTQD_Set2MeterSpd_flg]
  [VTQD_Set2MeterSpd_flg] -> ACCSetSpd_2506/6(VTQD_Set2MeterSpd_flg)
  VTQD_SetRoadSpdLim_flg/1 -> [VTQD_SetRoadSpdLim_flg]
  [VTQD_SetRoadSpdLim_flg] -> ACCSetSpd_2506/10(VTQD_SetRoadSpdLim_flg)
  VINP_ADASSLIFSpdLim_enum/1 -> [VINP_ADASSLIFSpdLim_enum]
  [VINP_ADASSLIFSpdLim_enum] -> Equal53/1
  VTQD_LScrollPressShort_flg/1 -> [VTQD_LScrollPressShort_flg]
  [VTQD_LScrollPressShort_flg] -> ACCSetSpd_2506/13(VTQD_LScrollPressShort_flg)
  VVMC_MeterIndSpeed_raw32/1 -> [VVMC_MeterIndSpeed_raw32]
  [VVMC_MeterIndSpeed_raw32] -> ACCSetSpd_2506/15(VVMC_MeterIndSpeed_raw32)
  Equal53/1 -> [VTQD_ADASSLIFSpdLimDet_flg]  "VTQD_ADASSLIFSpdLimDet_flg"
  [VTQD_ADASSLIFSpdLimDet_flg] -> ACCSetSpd_2506/12(VTQD_ADASSLIFSpdLimDet_flg)
  [VTQD_SWC2ScrollUpSta_flg] -> ACCSetSpd_2506/16(VTQD_SWC2ScrollUpSta_flg)
  [VTQD_SWC2ScrollDownSta_flg] -> ACCSetSpd_2506/17(VTQD_SWC2ScrollDownSta_flg)
  VTQD_SWC2ScrollDownSta_flg/1 -> [VTQD_SWC2ScrollDownSta_flg]
  VTQD_SWC2ScrollUpSta_flg/1 -> [VTQD_SWC2ScrollUpSta_flg]
  VTQD_LastSetSpd_kph/1 -> [VTQD_LastSetSpd_kph]
  [VTQD_LastSetSpd_kph] -> ACCSetSpd_2506/18(VTQD_LastSetSpd_kph)

== system tqd/TQD/TorqueDemand/Signal_convert/SWC2_Subsystem/Speed Setting Mode/CC Speed Setting ON ==
  note: CC SPEED SETTING MODE
  VVMC_CCCtrlSta_enum : Inport
  "VTQD_SWCResUpPress_enum  " : Inport  Port=2
  "VTQD_SWCSetDownPress_enum  " : Inport  Port=3
  VTQD_SpdLim4SetSpd_raw32 : Inport  Port=4
  VTQD_SetSpdDeltaLongFit_kph : Inport  Port=5
  VINP_Distanceunit_flg : Inport  Port=6
  VINP_SmartEcoModeSW_flg : Inport  Port=7
  Action Port : ActionPort  InitializeStates=reset
  " 1" : Constant  Value=KTQD_CCActiveMetSpdLo_kph
  " 2" : Constant  Value=KTQD_CCActiveMetSpdLoMPH_mph
  1 : Constant  Value=KTQD_SetSpdDeltaLongFit_kph
  2 : Constant  Value=KTQD_SetSpdDeltaShort_kph
  3 : Constant  Value=KTQD_CCActiveMetSpdHi_kph
  4 : Constant  Value=KTQD_SetSpdDeltaLong_kph
  5 : Constant  Value=KTQD_CCActiveMetSpdHiMPH_mph
  6 : Constant  Value=KTQD_SetSpdDeltaLongMPH_mph
  7 : Constant  Value=KTQD_SmartEcoLimitSpd_kph
  8 : Constant  Value=KTQD_SmartEcoLimitSpd_mph
  AND1 : Logic  AllPortsSameDT=off  OutDataTypeStr=boolean
  CC Speed Setting Mode : Stateflow chart  TreatAsAtomicUnit=on
      settings: PortSchema="{\"entries\":[{\"content\":{\"sides\":[{\"content\":{\"connectorIds\":[\"In5\",\"In12\",\"In4\",\"In3\",\"In9\",\"In6\",\"In7\",\"In8\",\"In1\",\"In2\",\"In11\",\"In10\"]},\"type\":\"ConnectorPlacement.EquallySpacedRectSide\",\"uuid\":\"331c8dfa-4564-419d-9323-fdbf8561d50b\"},{\"content\":{\"connectorIds\":[\"Out1\",\"Out2\"],\"side\":\"RIGHT\"},\"type\":\"ConnectorPlacement.EquallySpacedRectSide\",\"uuid\":\"71cb1444-7708-4b6f-91dd-d8a1c8c14ea8\"},{\"content\":{\"connectorIds\":[],\"side\":\"TOP\"},\"type\":\"ConnectorPlacement.EquallySpacedRectSide\",\"uuid\":\"6ecf38bb-d171-491a-a8b2-073f135e7039\"}]},\"type\":\"ConnectorPlacement.EquallySpacedConnector\",\"uuid\":\"fc3afa97-6e6e-4933-9aff-7c8f8cbb1702\"}],\"packageUris\":[\"http://schema.mathworks.com/mf0/Connector/R2020b\"],\"version\":\"1.0\"}"
  Cast To Single : DataTypeConversion  OutDataTypeStr=int8
  ONE : Constant  Value=ONE_INT
  Relational Operator2 : RelationalOperator  Operator===  OutDataTypeStr=boolean  RndMeth=Simplest
  Relational Operator4 : RelationalOperator  Operator===  OutDataTypeStr=boolean  RndMeth=Simplest
  Round : Rounding  Operator=round
  Specific_STATE_ChangeToSTANDBY : Stateflow chart  TreatAsAtomicUnit=on
  Switch{,1..5} (6 alike) : Switch  Criteria=u2 > Threshold
  standby : Constant  Value=ENUM_ADASCCSTA_STANDBY
  zero : Constant  Value=ZERO_INT
  VTQD_CCSetSpd_kph : Outport
  VTQD_SWC2CCSpdResetFinish_flg : Outport  Port=2
  wires:
  "VTQD_SWCSetDownPress_enum  "/1 -> CC Speed Setting Mode/10(VTQD_SWCSetDownPress_enum)
  [VTQD_ChangeToSTANDBY_flg] -> CC Speed Setting Mode/12(VTQD_ChangeToSTANDBY_flg)
  Specific_STATE_ChangeToSTANDBY/1(VTQD_CCChangeToSTANDBY_flg) -> [VTQD_ChangeToSTANDBY_flg]
  [VVMC_CCCtrlSta_enum] -> Specific_STATE_ChangeToSTANDBY/1(VVMC_CCCtrlSta_enum)
  "VTQD_SWCResUpPress_enum  "/1 -> CC Speed Setting Mode/11(VTQD_SWCResUpPress_enum)
  VVMC_CCCtrlSta_enum/1 -> CC Speed Setting Mode/5(VVMC_CCCtrlSta_enum), [VVMC_CCCtrlSta_enum]
  Switch2/1 -> CC Speed Setting Mode/7(KTQD_CCActiveMetSpdHi_raw32)
  2/1 -> CC Speed Setting Mode/2(KTQD_SetSpdDeltaShort_kph)
  Switch3/1 -> CC Speed Setting Mode/8(KTQD_CCActiveMetSpdLo_raw32)
  Switch4/1 -> CC Speed Setting Mode/1(KTQD_SetSpdDeltaLong_kph)
  CC Speed Setting Mode/2(VTQD_CCSpdResetFinish_flg) -> VTQD_SWC2CCSpdResetFinish_flg/1  "VTQD_SWC2CCSpdResetFinish_flg"
  VTQD_SetSpdDeltaLongFit_kph/1 -> CC Speed Setting Mode/4(VTQD_SetSpdDeltaLongFit_kph)
  1/1 -> CC Speed Setting Mode/3(KTQD_SetSpdDeltaLongFit_kph)
  VTQD_SpdLim4SetSpd_raw32/1 -> CC Speed Setting Mode/9(VVMC_MeterIndSpeed_raw32)
  Cast To Single/1 -> Relational Operator4/1, Switch1/3
  Switch1/1 -> VTQD_CCSetSpd_kph/1
  [VVMC_CCCtrlSta_enum] -> Relational Operator2/1
  AND1/1 -> Switch1/2
  ONE/1 -> Switch1/1
  standby/1 -> Relational Operator2/2
  zero/1 -> Relational Operator4/2
  Relational Operator2/1 -> AND1/1
  Relational Operator4/1 -> AND1/2
  [VINP_Distanceunit_flg] -> Switch2/2
  VINP_Distanceunit_flg/1 -> [VINP_Distanceunit_flg]
  [VINP_Distanceunit_flg] -> Switch3/2
  " 1"/1 -> Switch3/3
  " 2"/1 -> Switch3/1
  [VINP_Distanceunit_flg] -> Switch4/2
  4/1 -> Switch4/3
  6/1 -> Switch4/1
  [VINP_Distanceunit_flg] -> CC Speed Setting Mode/6(VINP_Distanceunit_flg)
  Round/1 -> Cast To Single/1
  CC Speed Setting Mode/1(VTQD_CCSetSpd_kph) -> Round/1
  VINP_SmartEcoModeSW_flg/1 -> [VINP_SmartEcoModeSW_flg]
  [VINP_SmartEcoModeSW_flg] -> Switch/2
  3/1 -> Switch/3
  Switch/1 -> Switch2/3
  5/1 -> Switch5/3
  [VINP_SmartEcoModeSW_flg] -> Switch5/2
  Switch5/1 -> Switch2/1
  8/1 -> Switch5/1
  7/1 -> Switch/1

== system tqd/TQD/TorqueDemand/Signal_convert/SWC2_Subsystem/Speed Setting Mode/Else Speed Setting On ==
  In : Inport
  Action Port : ActionPort
  Data Type Conversion : DataTypeConversion
  Out : Outport
  wires:
  Data Type Conversion/1 -> Out/1
  In/1 -> Data Type Conversion/1

== system tqd/TQD/TorqueDemand/Signal_convert/SWC2_Subsystem/Speed Setting Mode/ISA Speed Setting ON ==
  VINP_ADASSLIFSpdLim_enum : Inport
  VINP_SmartEcoModeSW_flg : Inport  Port=2
  Action Port : ActionPort
  8 : Constant  Value=KTQD_SmartEcoLimitSpd_kph
  Data Type Conversion : DataTypeConversion
  Min : MinMax  Inputs=2
  Switch : Switch  Criteria=u2 > Threshold
  VTQD_ISASetSpd_kph : Outport
  wires:
  Data Type Conversion/1 -> VTQD_ISASetSpd_kph/1
  VINP_SmartEcoModeSW_flg/1 -> Switch/2
  VINP_ADASSLIFSpdLim_enum/1 -> Min/2, Switch/3
  Min/1 -> Switch/1
  8/1 -> Min/1
  Switch/1 -> Data Type Conversion/1
